simulink model "fukt_test"  (R2023b)
settings: Solver=FixedStepAuto  StartTime=0.0  StopTime=inf  FixedStep=0.5  MaxStep=1  MinStep=1  RelTol=1e-3
undefined symbols (not defined in the file or in its folder): BOOL, DINT, OTL, slplc
libraries: arduinolib x3
(part 3 of 6)

== system fukt_test/PLC Controller Suite/__Logic/Fukt sampling/Fuktmätare sampling/__Logic/Variable Read ==
  __CoreVarRead : Subsystem  Tag=CoreVarReadBlock  DisableCoverage=on  TreatAsAtomicUnit=on  mask{PLCBlockType=CoreVarRead}
      mask init:
      | slplc.callbacks.initCoreVariable(gcb, 'read');
      mask Help: web([docroot '/plccoder/ref/__corevarread' '.html']);
      mask DialogControl PLCBlockTitle Prompt: Core Variable Read
  __Format : MATLAB Function  Tag=PLC_Format_Data  Priority=20  DisableCoverage=on  InitFcn=slplc.utils.setBlockAppearance('reset');  StopFcn=slplc.utils.setBlockAppearance('reset');  TreatAsAtomicUnit=on
  VarOut : Outport  VectorParamsAs1DForOutWhenUnconnected=off
  wires:
  __CoreVarRead/1(y) -> __Format/1(data), VarOut/1

== system fukt_test/PLC Controller Suite/__Logic/Fukt sampling/Fuktmätare sampling/__Logic/Variable Write ==
  VarIn : Inport
  VariableWriteEnableRead : Subsystem  DisableCoverage=on  TreatAsAtomicUnit=on  mask{PLCLabelTag=_Variable_Write_Enable, PLCBlockType=VariableWriteEnableRead}
      mask prompts: PLCLabelTag "Label Tag:"
      mask init:
      | block = gcb;
      | maskObj = Simulink.Mask.get(block);
      | maskObj.Display = sprintf('disp(''%s'');', PLCLabelTag);
      mask Help: web([docroot '/plccoder/ref/variablewriteenableread' '.html']);
      mask DialogControl PLCBlockTitle Prompt: Variable Write Enable Read
      mask Display: disp('_Variable_Write_Enable');
  __CoreVarRead : Subsystem  Tag=CoreVarReadBlock  DisableCoverage=on  TreatAsAtomicUnit=on  mask{PLCBlockType=CoreVarRead}
      mask init:
      | slplc.callbacks.initCoreVariable(gcb, 'read');
      mask Help: web([docroot '/plccoder/ref/__corevarread' '.html']);
      mask DialogControl PLCBlockTitle Prompt: Core Variable Read
  __Enable : Subsystem  Priority=12
  __Format : MATLAB Function  Tag=PLC_Format_Data  Priority=20  DisableCoverage=on  InitFcn=slplc.utils.setBlockAppearance('reset');  StopFcn=slplc.utils.setBlockAppearance('reset');  TreatAsAtomicUnit=on
  wires:
  VarIn/1 -> __Enable/1(VarIn)
  VariableWriteEnableRead/1(Out1) -> __Enable/Enable
  __CoreVarRead/1(y) -> __Format/1(data)

== system fukt_test/PLC Controller Suite/__Logic/Fukt sampling/Fuktmätare sampling/__Logic/XIC1 ==
  RungIn : Inport  PortDimensions=1
  BlockEnableRead : Subsystem  DisableCoverage=on  TreatAsAtomicUnit=on  mask{PLCLabelTag=_Block_Enable, PLCBlockType=BlockEnableRead}
      mask prompts: PLCLabelTag "Label Tag:"
      mask init:
      | block = gcb;
      | maskObj = Simulink.Mask.get(block);
      | maskObj.Display = sprintf('disp(''%s'');', PLCLabelTag);
      mask Help: web([docroot '/plccoder/ref/blockenableread' '.html']);
      mask DialogControl PLCBlockTitle Prompt: Block Enable Read
      mask Display: disp('_Block_Enable');
  Instruction_Enable : Subsystem  Priority=12  TreatAsAtomicUnit=on
  RungInOverride : Subsystem  DisableCoverage=on  TreatAsAtomicUnit=on
  __CoreVarRead : Subsystem  Tag=CoreVarReadBlock  DisableCoverage=on  TreatAsAtomicUnit=on  mask{PLCBlockType=CoreVarRead}
      mask init:
      | slplc.callbacks.initCoreVariable(gcb, 'read');
      mask Help: web([docroot '/plccoder/ref/__corevarread' '.html']);
      mask DialogControl PLCBlockTitle Prompt: Core Variable Read
  __Format : MATLAB Function  Tag=PLC_Format_Boolean  Priority=20  DisableCoverage=on  InitFcn=slplc.utils.setBlockAppearance('reset', '%<PLCOperandTag>');  StopFcn=slplc.utils.setBlockAppearance('reset', '%<PLCOperandTag>');  TreatAsAtomicUnit=on
  RungOut : Outport  OutDataTypeStr=BOOL  PortDimensions=1  InitialOutput=false  VectorParamsAs1DForOutWhenUnconnected=off
  wires:
  RungIn/1 -> RungInOverride/1(In1)
  Instruction_Enable/1(Rung-condition-out) -> __Format/3(RungOut), RungOut/1
  BlockEnableRead/1(Out1) -> __Format/1(BlockEnable), Instruction_Enable/Enable
  RungInOverride/1(Out1) -> __Format/2(RungIn), Instruction_Enable/1(Rung-condition-in)
  __CoreVarRead/1(y) -> __Format/4(data)  "DataBit"

== system fukt_test/PLC Controller Suite/__Logic/Fukt sampling/Fuktmätare sampling/__Logic/XIC2 ==
  RungIn : Inport  PortDimensions=1
  BlockEnableRead : Subsystem  DisableCoverage=on  TreatAsAtomicUnit=on  mask{PLCLabelTag=_Block_Enable, PLCBlockType=BlockEnableRead}
      mask prompts: PLCLabelTag "Label Tag:"
      mask init:
      | block = gcb;
      | maskObj = Simulink.Mask.get(block);
      | maskObj.Display = sprintf('disp(''%s'');', PLCLabelTag);
      mask Help: web([docroot '/plccoder/ref/blockenableread' '.html']);
      mask DialogControl PLCBlockTitle Prompt: Block Enable Read
      mask Display: disp('_Block_Enable');
  Instruction_Enable : Subsystem  Priority=12  TreatAsAtomicUnit=on
  RungInOverride : Subsystem  DisableCoverage=on  TreatAsAtomicUnit=on
  __CoreVarRead : Subsystem  Tag=CoreVarReadBlock  DisableCoverage=on  TreatAsAtomicUnit=on  mask{PLCBlockType=CoreVarRead}
      mask init:
      | slplc.callbacks.initCoreVariable(gcb, 'read');
      mask Help: web([docroot '/plccoder/ref/__corevarread' '.html']);
      mask DialogControl PLCBlockTitle Prompt: Core Variable Read
  __Format : MATLAB Function  Tag=PLC_Format_Boolean  Priority=20  DisableCoverage=on  InitFcn=slplc.utils.setBlockAppearance('reset', '%<PLCOperandTag>');  StopFcn=slplc.utils.setBlockAppearance('reset', '%<PLCOperandTag>');  TreatAsAtomicUnit=on
  RungOut : Outport  OutDataTypeStr=BOOL  PortDimensions=1  InitialOutput=false  VectorParamsAs1DForOutWhenUnconnected=off
  wires:
  __CoreVarRead/1(y) -> __Format/4(data)  "DataBit"
  RungInOverride/1(Out1) -> Instruction_Enable/1(Rung-condition-in), __Format/2(RungIn)
  BlockEnableRead/1(Out1) -> Instruction_Enable/Enable, __Format/1(BlockEnable)
  Instruction_Enable/1(Rung-condition-out) -> RungOut/1, __Format/3(RungOut)
  RungIn/1 -> RungInOverride/1(In1)

== system fukt_test/PLC Controller Suite/__Logic/Fukt logic/Program/__Logic/GEQ/BlockEnableRead ==
  __CoreLabelRead : Subsystem  Tag=CoreVarReadBlock  DisableCoverage=on  TreatAsAtomicUnit=on  mask{PLCBlockType=CoreLabelRead}
      mask init:
      | slplc.callbacks.initRoutineLabelRead(gcb);
      mask Help: web([docroot '/plccoder/ref/__corelabelread' '.html']);
      mask DialogControl PLCBlockTitle Prompt: Core Label Read
  Out1 : Outport  VectorParamsAs1DForOutWhenUnconnected=off
  wires:
  __CoreLabelRead/1(Out1) -> Out1/1

== system fukt_test/PLC Controller Suite/__Logic/Fukt logic/Program/__Logic/GEQ/Instruction_Enable ==
  Rung-condition-in : Inport
  srcA : Inport  Port=2  PortDimensions=1
  srcB : Inport  Port=3  PortDimensions=1
  Enable : EnablePort
  Logical Operator : Logic  OutDataTypeStr=BOOL
  Relational Operator : RelationalOperator  OutDataTypeStr=BOOL  RndMeth=Simplest  InputSameDT=off
  Rung-condition-out : Outport  PortDimensions=1  VectorParamsAs1DForOutWhenUnconnected=off
  wires:
  Rung-condition-in/1 -> Logical Operator/1
  srcB/1 -> Relational Operator/2
  srcA/1 -> Relational Operator/1
  Relational Operator/1 -> Logical Operator/2
  Logical Operator/1 -> Rung-condition-out/1  "Rung-condition-out"

== system fukt_test/PLC Controller Suite/__Logic/Fukt logic/Program/__Logic/GEQ/RungInOverride ==
  In1 : Inport
  AND : Logic  AllPortsSameDT=off  OutDataTypeStr=boolean
  ForceRungInFalseRead : Subsystem  DisableCoverage=on  TreatAsAtomicUnit=on  mask{PLCLabelTag=_Force_RungIn_False, PLCBlockType=ForceRungInFalseRead}
      mask prompts: PLCLabelTag "Label Tag:"
      mask init:
      | block = gcb;
      | maskObj = Simulink.Mask.get(block);
      | maskObj.Display = sprintf('disp(''%s'');', PLCLabelTag);
      mask Help: web([docroot '/plccoder/ref/forcerunginfalseread' '.html']);
      mask DialogControl PLCBlockTitle Prompt: Force Rung-In False Read
      mask Display: disp('_Force_RungIn_False');
  NOT : Logic  Operator=NOT  IconShape=distinctive  AllPortsSameDT=off  OutDataTypeStr=boolean
  Out1 : Outport  VectorParamsAs1DForOutWhenUnconnected=off
  wires:
  AND/1 -> Out1/1
  In1/1 -> AND/2
  ForceRungInFalseRead/1(Out1) -> NOT/1
  NOT/1 -> AND/1

== system fukt_test/PLC Controller Suite/__Logic/Fukt logic/Program/__Logic/OTL/BlockEnableRead ==
  __CoreLabelRead : Subsystem  Tag=CoreVarReadBlock  DisableCoverage=on  TreatAsAtomicUnit=on  mask{PLCBlockType=CoreLabelRead}
      mask init:
      | slplc.callbacks.initRoutineLabelRead(gcb);
      mask Help: web([docroot '/plccoder/ref/__corelabelread' '.html']);
      mask DialogControl PLCBlockTitle Prompt: Core Label Read
  Out1 : Outport  VectorParamsAs1DForOutWhenUnconnected=off
  wires:
  __CoreLabelRead/1(Out1) -> Out1/1

== system fukt_test/PLC Controller Suite/__Logic/Fukt logic/Program/__Logic/OTL/Instruction_Enable ==
  Rung-condition-in : Inport  OutDataTypeStr=BOOL
  Enable : EnablePort
  Rung-condition-in is true : Subsystem  Priority=12
  wires:
  Rung-condition-in/1 -> Rung-condition-in is true/Enable  "Rung-condition-in"

== system fukt_test/PLC Controller Suite/__Logic/Fukt logic/Program/__Logic/OTL/RungInOverride ==
  In1 : Inport
  AND : Logic  AllPortsSameDT=off  OutDataTypeStr=boolean
  ForceRungInFalseRead : Subsystem  DisableCoverage=on  TreatAsAtomicUnit=on  mask{PLCLabelTag=_Force_RungIn_False, PLCBlockType=ForceRungInFalseRead}
      mask prompts: PLCLabelTag "Label Tag:"
      mask init:
      | block = gcb;
      | maskObj = Simulink.Mask.get(block);
      | maskObj.Display = sprintf('disp(''%s'');', PLCLabelTag);
      mask Help: web([docroot '/plccoder/ref/forcerunginfalseread' '.html']);
      mask DialogControl PLCBlockTitle Prompt: Force Rung-In False Read
      mask Display: disp('_Force_RungIn_False');
  NOT : Logic  Operator=NOT  IconShape=distinctive  AllPortsSameDT=off  OutDataTypeStr=boolean
  Out1 : Outport  VectorParamsAs1DForOutWhenUnconnected=off
  wires:
  AND/1 -> Out1/1
  In1/1 -> AND/2
  ForceRungInFalseRead/1(Out1) -> NOT/1
  NOT/1 -> AND/1

== system fukt_test/PLC Controller Suite/__Logic/Fukt logic/Program/__Logic/OTL/__CoreVarRead ==
  DataRead : DataStoreRead  DataStoreName=xxx_PLC_VAR_OrangeLed  IndexOptions=Index vector (dialog)  Indices=1  OutputSizes=1
  y : Outport  VectorParamsAs1DForOutWhenUnconnected=off
  wires:
  DataRead/1 -> y/1

== system fukt_test/PLC Controller Suite/__Logic/Fukt logic/Program/__Logic/OTL1/BlockEnableRead ==
  __CoreLabelRead : Subsystem  Tag=CoreVarReadBlock  DisableCoverage=on  TreatAsAtomicUnit=on  mask{PLCBlockType=CoreLabelRead}
      mask init:
      | slplc.callbacks.initRoutineLabelRead(gcb);
      mask Help: web([docroot '/plccoder/ref/__corelabelread' '.html']);
      mask DialogControl PLCBlockTitle Prompt: Core Label Read
  Out1 : Outport  VectorParamsAs1DForOutWhenUnconnected=off
  wires:
  __CoreLabelRead/1(Out1) -> Out1/1

== system fukt_test/PLC Controller Suite/__Logic/Fukt logic/Program/__Logic/OTL1/Instruction_Enable ==
  Rung-condition-in : Inport  OutDataTypeStr=BOOL
  Enable : EnablePort
  Rung-condition-in is true : Subsystem  Priority=12
  wires:
  Rung-condition-in/1 -> Rung-condition-in is true/Enable  "Rung-condition-in"

== system fukt_test/PLC Controller Suite/__Logic/Fukt logic/Program/__Logic/OTL1/RungInOverride ==
  In1 : Inport
  AND : Logic  AllPortsSameDT=off  OutDataTypeStr=boolean
  ForceRungInFalseRead : Subsystem  DisableCoverage=on  TreatAsAtomicUnit=on  mask{PLCLabelTag=_Force_RungIn_False, PLCBlockType=ForceRungInFalseRead}
      mask prompts: PLCLabelTag "Label Tag:"
      mask init:
      | block = gcb;
      | maskObj = Simulink.Mask.get(block);
      | maskObj.Display = sprintf('disp(''%s'');', PLCLabelTag);
      mask Help: web([docroot '/plccoder/ref/forcerunginfalseread' '.html']);
      mask DialogControl PLCBlockTitle Prompt: Force Rung-In False Read
      mask Display: disp('_Force_RungIn_False');
  NOT : Logic  Operator=NOT  IconShape=distinctive  AllPortsSameDT=off  OutDataTypeStr=boolean
  Out1 : Outport  VectorParamsAs1DForOutWhenUnconnected=off
  wires:
  AND/1 -> Out1/1
  In1/1 -> AND/2
  ForceRungInFalseRead/1(Out1) -> NOT/1
  NOT/1 -> AND/1

== system fukt_test/PLC Controller Suite/__Logic/Fukt logic/Program/__Logic/OTL1/__CoreVarRead ==
  DataRead : DataStoreRead  DataStoreName=xxx_PLC_VAR_fukt_bool  IndexOptions=Index vector (dialog)  Indices=1  OutputSizes=1
  y : Outport  VectorParamsAs1DForOutWhenUnconnected=off
  wires:
  DataRead/1 -> y/1

== system fukt_test/PLC Controller Suite/__Logic/Fukt logic/Program/__Logic/OTU/BlockEnableRead ==
  __CoreLabelRead : Subsystem  Tag=CoreVarReadBlock  DisableCoverage=on  TreatAsAtomicUnit=on  mask{PLCBlockType=CoreLabelRead}
      mask init:
      | slplc.callbacks.initRoutineLabelRead(gcb);
      mask Help: web([docroot '/plccoder/ref/__corelabelread' '.html']);
      mask DialogControl PLCBlockTitle Prompt: Core Label Read
  Out1 : Outport  VectorParamsAs1DForOutWhenUnconnected=off
  wires:
  __CoreLabelRead/1(Out1) -> Out1/1

== system fukt_test/PLC Controller Suite/__Logic/Fukt logic/Program/__Logic/OTU/Instruction_Enable ==
  Rung-condition-in : Inport  OutDataTypeStr=BOOL
  Enable : EnablePort
  Rung-condition-in is true : Subsystem  Priority=12
  wires:
  Rung-condition-in/1 -> Rung-condition-in is true/Enable  "Rung-condition-in"

== system fukt_test/PLC Controller Suite/__Logic/Fukt logic/Program/__Logic/OTU/RungInOverride ==
  In1 : Inport
  AND : Logic  AllPortsSameDT=off  OutDataTypeStr=boolean
  ForceRungInFalseRead : Subsystem  DisableCoverage=on  TreatAsAtomicUnit=on  mask{PLCLabelTag=_Force_RungIn_False, PLCBlockType=ForceRungInFalseRead}
      mask prompts: PLCLabelTag "Label Tag:"
      mask init:
      | block = gcb;
      | maskObj = Simulink.Mask.get(block);
      | maskObj.Display = sprintf('disp(''%s'');', PLCLabelTag);
      mask Help: web([docroot '/plccoder/ref/forcerunginfalseread' '.html']);
      mask DialogControl PLCBlockTitle Prompt: Force Rung-In False Read
      mask Display: disp('_Force_RungIn_False');
  NOT : Logic  Operator=NOT  IconShape=distinctive  AllPortsSameDT=off  OutDataTypeStr=boolean
  Out1 : Outport  VectorParamsAs1DForOutWhenUnconnected=off
  wires:
  AND/1 -> Out1/1
  In1/1 -> AND/2
  ForceRungInFalseRead/1(Out1) -> NOT/1
  NOT/1 -> AND/1

== system fukt_test/PLC Controller Suite/__Logic/Fukt logic/Program/__Logic/OTU/__CoreVarRead ==
  DataRead : DataStoreRead  DataStoreName=xxx_PLC_VAR_OrangeLed  IndexOptions=Index vector (dialog)  Indices=1  OutputSizes=1
  y : Outport  VectorParamsAs1DForOutWhenUnconnected=off
  wires:
  DataRead/1 -> y/1

== system fukt_test/PLC Controller Suite/__Logic/Fukt logic/Program/__Logic/OTU1/BlockEnableRead ==
  __CoreLabelRead : Subsystem  Tag=CoreVarReadBlock  DisableCoverage=on  TreatAsAtomicUnit=on  mask{PLCBlockType=CoreLabelRead}
      mask init:
      | slplc.callbacks.initRoutineLabelRead(gcb);
      mask Help: web([docroot '/plccoder/ref/__corelabelread' '.html']);
      mask DialogControl PLCBlockTitle Prompt: Core Label Read
  Out1 : Outport  VectorParamsAs1DForOutWhenUnconnected=off
  wires:
  __CoreLabelRead/1(Out1) -> Out1/1

== system fukt_test/PLC Controller Suite/__Logic/Fukt logic/Program/__Logic/OTU1/Instruction_Enable ==
  Rung-condition-in : Inport  OutDataTypeStr=BOOL
  Enable : EnablePort
  Rung-condition-in is true : Subsystem  Priority=12
  wires:
  Rung-condition-in/1 -> Rung-condition-in is true/Enable  "Rung-condition-in"

== system fukt_test/PLC Controller Suite/__Logic/Fukt logic/Program/__Logic/OTU1/RungInOverride ==
  In1 : Inport
  AND : Logic  AllPortsSameDT=off  OutDataTypeStr=boolean
  ForceRungInFalseRead : Subsystem  DisableCoverage=on  TreatAsAtomicUnit=on  mask{PLCLabelTag=_Force_RungIn_False, PLCBlockType=ForceRungInFalseRead}
      mask prompts: PLCLabelTag "Label Tag:"
      mask init:
      | block = gcb;
      | maskObj = Simulink.Mask.get(block);
      | maskObj.Display = sprintf('disp(''%s'');', PLCLabelTag);
      mask Help: web([docroot '/plccoder/ref/forcerunginfalseread' '.html']);
      mask DialogControl PLCBlockTitle Prompt: Force Rung-In False Read
      mask Display: disp('_Force_RungIn_False');
  NOT : Logic  Operator=NOT  IconShape=distinctive  AllPortsSameDT=off  OutDataTypeStr=boolean
  Out1 : Outport  VectorParamsAs1DForOutWhenUnconnected=off
  wires:
  AND/1 -> Out1/1
  In1/1 -> AND/2
  ForceRungInFalseRead/1(Out1) -> NOT/1
  NOT/1 -> AND/1

== system fukt_test/PLC Controller Suite/__Logic/Fukt logic/Program/__Logic/OTU1/__CoreVarRead ==
  DataRead : DataStoreRead  DataStoreName=xxx_PLC_VAR_fukt_polling  IndexOptions=Index vector (dialog)  Indices=1  OutputSizes=1
  y : Outport  VectorParamsAs1DForOutWhenUnconnected=off
  wires:
  DataRead/1 -> y/1

== system fukt_test/PLC Controller Suite/__Logic/Fukt logic/Program/__Logic/OTU2/BlockEnableRead ==
  __CoreLabelRead : Subsystem  Tag=CoreVarReadBlock  DisableCoverage=on  TreatAsAtomicUnit=on  mask{PLCBlockType=CoreLabelRead}
      mask init:
      | slplc.callbacks.initRoutineLabelRead(gcb);
      mask Help: web([docroot '/plccoder/ref/__corelabelread' '.html']);
      mask DialogControl PLCBlockTitle Prompt: Core Label Read
  Out1 : Outport  VectorParamsAs1DForOutWhenUnconnected=off
  wires:
  __CoreLabelRead/1(Out1) -> Out1/1

== system fukt_test/PLC Controller Suite/__Logic/Fukt logic/Program/__Logic/OTU2/Instruction_Enable ==
  Rung-condition-in : Inport  OutDataTypeStr=BOOL
  Enable : EnablePort
  Rung-condition-in is true : Subsystem  Priority=12
  wires:
  Rung-condition-in/1 -> Rung-condition-in is true/Enable  "Rung-condition-in"

== system fukt_test/PLC Controller Suite/__Logic/Fukt logic/Program/__Logic/OTU2/RungInOverride ==
  In1 : Inport
  AND : Logic  AllPortsSameDT=off  OutDataTypeStr=boolean
  ForceRungInFalseRead : Subsystem  DisableCoverage=on  TreatAsAtomicUnit=on  mask{PLCLabelTag=_Force_RungIn_False, PLCBlockType=ForceRungInFalseRead}
      mask prompts: PLCLabelTag "Label Tag:"
      mask init:
      | block = gcb;
      | maskObj = Simulink.Mask.get(block);
      | maskObj.Display = sprintf('disp(''%s'');', PLCLabelTag);
      mask Help: web([docroot '/plccoder/ref/forcerunginfalseread' '.html']);
      mask DialogControl PLCBlockTitle Prompt: Force Rung-In False Read
      mask Display: disp('_Force_RungIn_False');
  NOT : Logic  Operator=NOT  IconShape=distinctive  AllPortsSameDT=off  OutDataTypeStr=boolean
  Out1 : Outport  VectorParamsAs1DForOutWhenUnconnected=off
  wires:
  AND/1 -> Out1/1
  In1/1 -> AND/2
  ForceRungInFalseRead/1(Out1) -> NOT/1
  NOT/1 -> AND/1

== system fukt_test/PLC Controller Suite/__Logic/Fukt logic/Program/__Logic/OTU2/__CoreVarRead ==
  DataRead : DataStoreRead  DataStoreName=xxx_PLC_VAR_fukt_bool  IndexOptions=Index vector (dialog)  Indices=1  OutputSizes=1
  y : Outport  VectorParamsAs1DForOutWhenUnconnected=off
  wires:
  DataRead/1 -> y/1

== system fukt_test/PLC Controller Suite/__Logic/Fukt logic/Program/__Logic/TON/BlockEnableRead ==
  __CoreLabelRead : Subsystem  Tag=CoreVarReadBlock  DisableCoverage=on  TreatAsAtomicUnit=on  mask{PLCBlockType=CoreLabelRead}
      mask init:
      | slplc.callbacks.initRoutineLabelRead(gcb);
      mask Help: web([docroot '/plccoder/ref/__corelabelread' '.html']);
      mask DialogControl PLCBlockTitle Prompt: Core Label Read
  Out1 : Outport  VectorParamsAs1DForOutWhenUnconnected=off
  wires:
  __CoreLabelRead/1(Out1) -> Out1/1

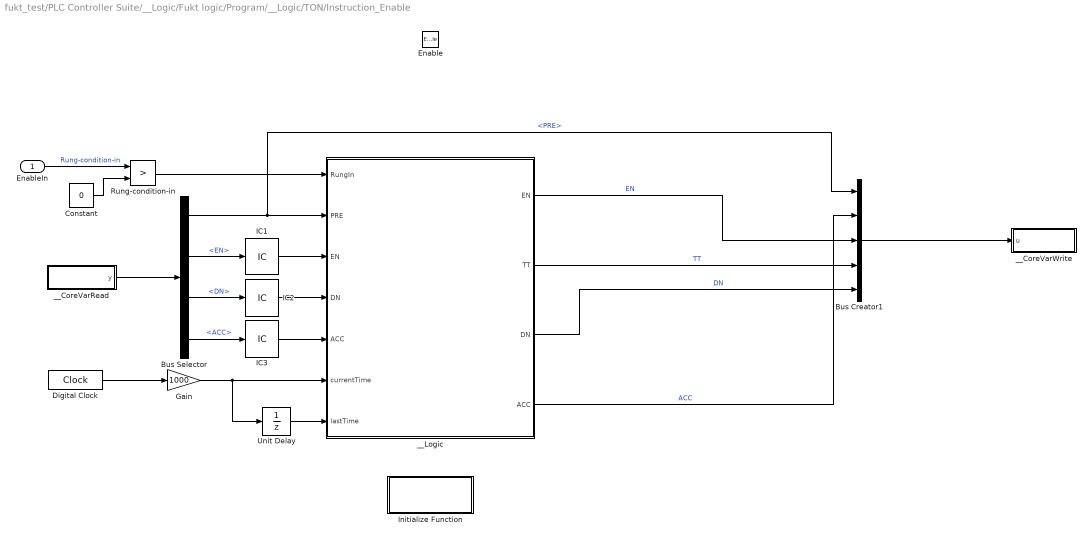
== system fukt_test/PLC Controller Suite/__Logic/Fukt logic/Program/__Logic/TON/Instruction_Enable ==
  EnableIn : Inport
  Enable : EnablePort
  Bus Creator1 : BusCreator  Inputs=5  OutDataTypeStr=Bus: TIMER  NonVirtualBus=on
  Bus Selector : BusSelector  OutputSignals=PRE,EN,DN,ACC
  Constant : Constant  Value=0
  Digital Clock : DigitalClock  SampleTime=PLCTimerSampleTime
  Gain : Gain  Gain=1000
  IC1 : InitialCondition  Value=false
  IC2 : InitialCondition  Value=false
  IC3 : InitialCondition  Value=0
  Initialize Function : Subsystem  TreatAsAtomicUnit=on
  Rung-condition-in : RelationalOperator  Operator=>  OutDataTypeStr=boolean  RndMeth=Simplest  InputSameDT=off
  Unit Delay : UnitDelay  SampleTime=-1  HasFrameUpgradeWarning=on
  __CoreVarRead : Subsystem  Tag=CoreVarReadBlock  DisableCoverage=on  TreatAsAtomicUnit=on  mask{PLCBlockType=CoreVarRead}
      mask init:
      | slplc.callbacks.initCoreVariable(gcb, 'read');
      mask Help: web([docroot '/plccoder/ref/__corevarread' '.html']);
      mask DialogControl PLCBlockTitle Prompt: Core Variable Read
  __CoreVarWrite : Subsystem  Tag=CoreVarWriteBlock  DisableCoverage=on  TreatAsAtomicUnit=on  mask{PLCBlockType=CoreVarWrite}
      mask init:
      | slplc.callbacks.initCoreVariable(gcb, 'write');
      mask Help: web([docroot '/plccoder/ref/__corevarwrite' '.html']);
      mask DialogControl PLCBlockTitle Prompt: Core Variable Write
  __Logic : MATLAB Function  Priority=12  DisableCoverage=on
  wires:
  IC3/1 -> __Logic/5("ACC ")
  IC2/1 -> __Logic/4("DN ")
  IC1/1 -> __Logic/3("EN ")
  Rung-condition-in/1 -> __Logic/1(RungIn)
  Bus Selector/2 -> IC1/1  "<EN>"
  Gain/1 -> __Logic/6(currentTime), Unit Delay/1
  Bus Selector/3 -> IC2/1  "<DN>"
  __CoreVarRead/1(y) -> Bus Selector/1
  Unit Delay/1 -> __Logic/7(lastTime)
  Bus Creator1/1 -> __CoreVarWrite/1(u)
  __Logic/4(ACC) -> Bus Creator1/2  "ACC"
  __Logic/3(DN) -> Bus Creator1/5  "DN"
  Digital Clock/1 -> Gain/1
  EnableIn/1 -> Rung-condition-in/1  "Rung-condition-in"
  Bus Selector/1 -> Bus Creator1/1, __Logic/2(PRE)  "<PRE>"
  __Logic/2(TT) -> Bus Creator1/4  "TT"
  Bus Selector/4 -> IC3/1  "<ACC>"
  __Logic/1(EN) -> Bus Creator1/3  "EN"
  Constant/1 -> Rung-condition-in/2

== system fukt_test/PLC Controller Suite/__Logic/Fukt logic/Program/__Logic/TON/RungInOverride ==
  In1 : Inport
  AND : Logic  AllPortsSameDT=off  OutDataTypeStr=boolean
  ForceRungInFalseRead : Subsystem  DisableCoverage=on  TreatAsAtomicUnit=on  mask{PLCLabelTag=_Force_RungIn_False, PLCBlockType=ForceRungInFalseRead}
      mask prompts: PLCLabelTag "Label Tag:"
      mask init:
      | block = gcb;
      | maskObj = Simulink.Mask.get(block);
      | maskObj.Display = sprintf('disp(''%s'');', PLCLabelTag);
      mask Help: web([docroot '/plccoder/ref/forcerunginfalseread' '.html']);
      mask DialogControl PLCBlockTitle Prompt: Force Rung-In False Read
      mask Display: disp('_Force_RungIn_False');
  NOT : Logic  Operator=NOT  IconShape=distinctive  AllPortsSameDT=off  OutDataTypeStr=boolean
  Out1 : Outport  VectorParamsAs1DForOutWhenUnconnected=off
  wires:
  AND/1 -> Out1/1
  In1/1 -> AND/2
  ForceRungInFalseRead/1(Out1) -> NOT/1
  NOT/1 -> AND/1

== system fukt_test/PLC Controller Suite/__Logic/Fukt logic/Program/__Logic/TON/__CoreVarRead ==
  DataRead : DataStoreRead  DataStoreName=xxx_PLC_VAR_orange_led_timer_1  IndexOptions=Index vector (dialog)  Indices=1  OutputSizes=1
  y : Outport  VectorParamsAs1DForOutWhenUnconnected=off
  wires:
  DataRead/1 -> y/1

== system fukt_test/PLC Controller Suite/__Logic/Fukt logic/Program/__Logic/Variable Read/__CoreVarRead ==
  DataRead : DataStoreRead  DataStoreName=xxx_PLC_VAR_Fukt_value_copy  IndexOptions=Index vector (dialog)  Indices=1  OutputSizes=1
  y : Outport  VectorParamsAs1DForOutWhenUnconnected=off
  wires:
  DataRead/1 -> y/1

== system fukt_test/PLC Controller Suite/__Logic/Fukt logic/Program/__Logic/Variable Read1/__CoreVarRead ==
  DataRead : DataStoreRead  DataStoreName=xxx_PLC_VAR_Fukt_constant  IndexOptions=Index vector (dialog)  Indices=1  OutputSizes=1
  y : Outport  VectorParamsAs1DForOutWhenUnconnected=off
  wires:
  DataRead/1 -> y/1

== system fukt_test/PLC Controller Suite/__Logic/Fukt logic/Program/__Logic/XIC1/BlockEnableRead ==
  __CoreLabelRead : Subsystem  Tag=CoreVarReadBlock  DisableCoverage=on  TreatAsAtomicUnit=on  mask{PLCBlockType=CoreLabelRead}
      mask init:
      | slplc.callbacks.initRoutineLabelRead(gcb);
      mask Help: web([docroot '/plccoder/ref/__corelabelread' '.html']);
      mask DialogControl PLCBlockTitle Prompt: Core Label Read
  Out1 : Outport  VectorParamsAs1DForOutWhenUnconnected=off
  wires:
  __CoreLabelRead/1(Out1) -> Out1/1

== system fukt_test/PLC Controller Suite/__Logic/Fukt logic/Program/__Logic/XIC1/Instruction_Enable ==
  Rung-condition-in : Inport  OutDataTypeStr=BOOL
  Enable : EnablePort
  Logical Operator : Logic  OutDataTypeStr=BOOL
  __CoreVarRead : Subsystem  Tag=CoreVarReadBlock  DisableCoverage=on  TreatAsAtomicUnit=on  mask{PLCBlockType=CoreVarRead}
      mask init:
      | slplc.callbacks.initCoreVariable(gcb, 'read');
      mask Help: web([docroot '/plccoder/ref/__corevarread' '.html']);
      mask DialogControl PLCBlockTitle Prompt: Core Variable Read
  Rung-condition-out : Outport  VectorParamsAs1DForOutWhenUnconnected=off
  wires:
  Rung-condition-in/1 -> Logical Operator/1  "Rung-condition-in"
  Logical Operator/1 -> Rung-condition-out/1  "Rung-condition-out"
  __CoreVarRead/1(y) -> Logical Operator/2  "DataBit"

== system fukt_test/PLC Controller Suite/__Logic/Fukt logic/Program/__Logic/XIC1/RungInOverride ==
  In1 : Inport
  AND : Logic  AllPortsSameDT=off  OutDataTypeStr=boolean
  ForceRungInFalseRead : Subsystem  DisableCoverage=on  TreatAsAtomicUnit=on  mask{PLCLabelTag=_Force_RungIn_False, PLCBlockType=ForceRungInFalseRead}
      mask prompts: PLCLabelTag "Label Tag:"
      mask init:
      | block = gcb;
      | maskObj = Simulink.Mask.get(block);
      | maskObj.Display = sprintf('disp(''%s'');', PLCLabelTag);
      mask Help: web([docroot '/plccoder/ref/forcerunginfalseread' '.html']);
      mask DialogControl PLCBlockTitle Prompt: Force Rung-In False Read
      mask Display: disp('_Force_RungIn_False');
  NOT : Logic  Operator=NOT  IconShape=distinctive  AllPortsSameDT=off  OutDataTypeStr=boolean
  Out1 : Outport  VectorParamsAs1DForOutWhenUnconnected=off
  wires:
  AND/1 -> Out1/1
  In1/1 -> AND/2
  ForceRungInFalseRead/1(Out1) -> NOT/1
  NOT/1 -> AND/1

== system fukt_test/PLC Controller Suite/__Logic/Fukt logic/Program/__Logic/XIC1/__CoreVarRead ==
  DataRead : DataStoreRead  DataStoreName=xxx_PLC_VAR_orange_led_timer_1  DataStoreElements=xxx_PLC_VAR_orange_led_timer_1.DN  IndexOptions=Index vector (dialog)  Indices=1  OutputSizes=1
  y : Outport  VectorParamsAs1DForOutWhenUnconnected=off
  wires:
  DataRead/1 -> y/1

== system fukt_test/PLC Controller Suite/__Logic/Fukt logic/Program/__Logic/XIC2/BlockEnableRead ==
  __CoreLabelRead : Subsystem  Tag=CoreVarReadBlock  DisableCoverage=on  TreatAsAtomicUnit=on  mask{PLCBlockType=CoreLabelRead}
      mask init:
      | slplc.callbacks.initRoutineLabelRead(gcb);
      mask Help: web([docroot '/plccoder/ref/__corelabelread' '.html']);
      mask DialogControl PLCBlockTitle Prompt: Core Label Read
  Out1 : Outport  VectorParamsAs1DForOutWhenUnconnected=off
  wires:
  __CoreLabelRead/1(Out1) -> Out1/1

== system fukt_test/PLC Controller Suite/__Logic/Fukt logic/Program/__Logic/XIC2/Instruction_Enable ==
  Rung-condition-in : Inport  OutDataTypeStr=BOOL
  Enable : EnablePort
  Logical Operator : Logic  OutDataTypeStr=BOOL
  __CoreVarRead : Subsystem  Tag=CoreVarReadBlock  DisableCoverage=on  TreatAsAtomicUnit=on  mask{PLCBlockType=CoreVarRead}
      mask init:
      | slplc.callbacks.initCoreVariable(gcb, 'read');
      mask Help: web([docroot '/plccoder/ref/__corevarread' '.html']);
      mask DialogControl PLCBlockTitle Prompt: Core Variable Read
  Rung-condition-out : Outport  VectorParamsAs1DForOutWhenUnconnected=off
  wires:
  __CoreVarRead/1(y) -> Logical Operator/2  "DataBit"
  Logical Operator/1 -> Rung-condition-out/1  "Rung-condition-out"
  Rung-condition-in/1 -> Logical Operator/1  "Rung-condition-in"

== system fukt_test/PLC Controller Suite/__Logic/Fukt logic/Program/__Logic/XIC2/RungInOverride ==
  In1 : Inport
  AND : Logic  AllPortsSameDT=off  OutDataTypeStr=boolean
  ForceRungInFalseRead : Subsystem  DisableCoverage=on  TreatAsAtomicUnit=on  mask{PLCLabelTag=_Force_RungIn_False, PLCBlockType=ForceRungInFalseRead}
      mask prompts: PLCLabelTag "Label Tag:"
      mask init:
      | block = gcb;
      | maskObj = Simulink.Mask.get(block);
      | maskObj.Display = sprintf('disp(''%s'');', PLCLabelTag);
      mask Help: web([docroot '/plccoder/ref/forcerunginfalseread' '.html']);
      mask DialogControl PLCBlockTitle Prompt: Force Rung-In False Read
      mask Display: disp('_Force_RungIn_False');
  NOT : Logic  Operator=NOT  IconShape=distinctive  AllPortsSameDT=off  OutDataTypeStr=boolean
  Out1 : Outport  VectorParamsAs1DForOutWhenUnconnected=off
  wires:
  NOT/1 -> AND/1
  ForceRungInFalseRead/1(Out1) -> NOT/1
  In1/1 -> AND/2
  AND/1 -> Out1/1

== system fukt_test/PLC Controller Suite/__Logic/Fukt logic/Program/__Logic/XIC2/__CoreVarRead ==
  DataRead : DataStoreRead  DataStoreName=xxx_PLC_VAR_fukt_polling  IndexOptions=Index vector (dialog)  Indices=1  OutputSizes=1
  y : Outport  VectorParamsAs1DForOutWhenUnconnected=off
  wires:
  DataRead/1 -> y/1

== system fukt_test/PLC Controller Suite/__Logic/Fukt logic/Program/__Logic/XIC3/BlockEnableRead ==
  __CoreLabelRead : Subsystem  Tag=CoreVarReadBlock  DisableCoverage=on  TreatAsAtomicUnit=on  mask{PLCBlockType=CoreLabelRead}
      mask init:
      | slplc.callbacks.initRoutineLabelRead(gcb);
      mask Help: web([docroot '/plccoder/ref/__corelabelread' '.html']);
      mask DialogControl PLCBlockTitle Prompt: Core Label Read
  Out1 : Outport  VectorParamsAs1DForOutWhenUnconnected=off
  wires:
  __CoreLabelRead/1(Out1) -> Out1/1

== system fukt_test/PLC Controller Suite/__Logic/Fukt logic/Program/__Logic/XIC3/Instruction_Enable ==
  Rung-condition-in : Inport  OutDataTypeStr=BOOL
  Enable : EnablePort
  Logical Operator : Logic  OutDataTypeStr=BOOL
  __CoreVarRead : Subsystem  Tag=CoreVarReadBlock  DisableCoverage=on  TreatAsAtomicUnit=on  mask{PLCBlockType=CoreVarRead}
      mask init:
      | slplc.callbacks.initCoreVariable(gcb, 'read');
      mask Help: web([docroot '/plccoder/ref/__corevarread' '.html']);
      mask DialogControl PLCBlockTitle Prompt: Core Variable Read
  Rung-condition-out : Outport  VectorParamsAs1DForOutWhenUnconnected=off
  wires:
  Rung-condition-in/1 -> Logical Operator/1  "Rung-condition-in"
  Logical Operator/1 -> Rung-condition-out/1  "Rung-condition-out"
  __CoreVarRead/1(y) -> Logical Operator/2  "DataBit"

== system fukt_test/PLC Controller Suite/__Logic/Fukt logic/Program/__Logic/XIC3/RungInOverride ==
  In1 : Inport
  AND : Logic  AllPortsSameDT=off  OutDataTypeStr=boolean
  ForceRungInFalseRead : Subsystem  DisableCoverage=on  TreatAsAtomicUnit=on  mask{PLCLabelTag=_Force_RungIn_False, PLCBlockType=ForceRungInFalseRead}
      mask prompts: PLCLabelTag "Label Tag:"
      mask init:
      | block = gcb;
      | maskObj = Simulink.Mask.get(block);
      | maskObj.Display = sprintf('disp(''%s'');', PLCLabelTag);
      mask Help: web([docroot '/plccoder/ref/forcerunginfalseread' '.html']);
      mask DialogControl PLCBlockTitle Prompt: Force Rung-In False Read
      mask Display: disp('_Force_RungIn_False');
  NOT : Logic  Operator=NOT  IconShape=distinctive  AllPortsSameDT=off  OutDataTypeStr=boolean
  Out1 : Outport  VectorParamsAs1DForOutWhenUnconnected=off
  wires:
  AND/1 -> Out1/1
  In1/1 -> AND/2
  ForceRungInFalseRead/1(Out1) -> NOT/1
  NOT/1 -> AND/1

== system fukt_test/PLC Controller Suite/__Logic/Fukt logic/Program/__Logic/XIC3/__CoreVarRead ==
  DataRead : DataStoreRead  DataStoreName=xxx_PLC_VAR_fukt_bool  IndexOptions=Index vector (dialog)  Indices=1  OutputSizes=1
  y : Outport  VectorParamsAs1DForOutWhenUnconnected=off
  wires:
  DataRead/1 -> y/1

== system fukt_test/PLC Controller Suite/__Logic/Fukt sampling/Fuktmätare sampling/__Logic/MOV/BlockEnableRead ==
  __CoreLabelRead : Subsystem  Tag=CoreVarReadBlock  DisableCoverage=on  TreatAsAtomicUnit=on  mask{PLCBlockType=CoreLabelRead}
      mask init:
      | slplc.callbacks.initRoutineLabelRead(gcb);
      mask Help: web([docroot '/plccoder/ref/__corelabelread' '.html']);
      mask DialogControl PLCBlockTitle Prompt: Core Label Read
  Out1 : Outport  VectorParamsAs1DForOutWhenUnconnected=off
  wires:
  __CoreLabelRead/1(Out1) -> Out1/1

== system fukt_test/PLC Controller Suite/__Logic/Fukt sampling/Fuktmätare sampling/__Logic/MOV/Instruction_Enable ==
  src : Inport  PortDimensions=1
  Enable : EnablePort
  Data Type Conversion : DataTypeConversion  RndMeth=Convergent  SaturateOnIntegerOverflow=off
  dest : Outport  PortDimensions=1  VectorParamsAs1DForOutWhenUnconnected=off
  wires:
  Data Type Conversion/1 -> dest/1
  src/1 -> Data Type Conversion/1

== system fukt_test/PLC Controller Suite/__Logic/Fukt sampling/Fuktmätare sampling/__Logic/MOV/RungInOverride ==
  In1 : Inport
  AND : Logic  AllPortsSameDT=off  OutDataTypeStr=boolean
  ForceRungInFalseRead : Subsystem  DisableCoverage=on  TreatAsAtomicUnit=on  mask{PLCLabelTag=_Force_RungIn_False, PLCBlockType=ForceRungInFalseRead}
      mask prompts: PLCLabelTag "Label Tag:"
      mask init:
      | block = gcb;
      | maskObj = Simulink.Mask.get(block);
      | maskObj.Display = sprintf('disp(''%s'');', PLCLabelTag);
      mask Help: web([docroot '/plccoder/ref/forcerunginfalseread' '.html']);
      mask DialogControl PLCBlockTitle Prompt: Force Rung-In False Read
      mask Display: disp('_Force_RungIn_False');
  NOT : Logic  Operator=NOT  IconShape=distinctive  AllPortsSameDT=off  OutDataTypeStr=boolean
  Out1 : Outport  VectorParamsAs1DForOutWhenUnconnected=off
  wires:
  AND/1 -> Out1/1
  In1/1 -> AND/2
  ForceRungInFalseRead/1(Out1) -> NOT/1
  NOT/1 -> AND/1

== system fukt_test/PLC Controller Suite/__Logic/Fukt sampling/Fuktmätare sampling/__Logic/MOV/RungOutOverride ==
  In1 : Inport
  AND : Logic  AllPortsSameDT=off  OutDataTypeStr=boolean
  BlockEnableRead : Subsystem  DisableCoverage=on  TreatAsAtomicUnit=on  mask{PLCLabelTag=_Block_Enable, PLCBlockType=BlockEnableRead}
      mask prompts: PLCLabelTag "Label Tag:"
      mask init:
      | block = gcb;
      | maskObj = Simulink.Mask.get(block);
      | maskObj.Display = sprintf('disp(''%s'');', PLCLabelTag);
      mask Help: web([docroot '/plccoder/ref/blockenableread' '.html']);
      mask DialogControl PLCBlockTitle Prompt: Block Enable Read
      mask Display: disp('_Block_Enable');
  VariableWriteEnableWrite : Subsystem  DisableCoverage=on  TreatAsAtomicUnit=on  mask{PLCLabelTag=_Variable_Write_Enable, PLCBlockType=VariableWriteEnableWrite}
      mask prompts: PLCLabelTag "Label Tag:"
      mask init:
      | block = gcb;
      | maskObj = Simulink.Mask.get(block);
      | maskObj.Display = sprintf('disp(''%s'');', PLCLabelTag);
      mask Help: web([docroot '/plccoder/ref/variablewriteenablewrite' '.html']);
      mask DialogControl PLCBlockTitle Prompt: Variable Write_Enable_Write
      mask Display: disp('_Variable_Write_Enable');
  Out1 : Outport  VectorParamsAs1DForOutWhenUnconnected=off
  wires:
  AND/1 -> VariableWriteEnableWrite/1(In1), Out1/1
  BlockEnableRead/1(Out1) -> AND/1
  In1/1 -> AND/2

== system fukt_test/PLC Controller Suite/__Logic/Fukt sampling/Fuktmätare sampling/__Logic/OTL/BlockEnableRead ==
  __CoreLabelRead : Subsystem  Tag=CoreVarReadBlock  DisableCoverage=on  TreatAsAtomicUnit=on  mask{PLCBlockType=CoreLabelRead}
      mask init:
      | slplc.callbacks.initRoutineLabelRead(gcb);
      mask Help: web([docroot '/plccoder/ref/__corelabelread' '.html']);
      mask DialogControl PLCBlockTitle Prompt: Core Label Read
  Out1 : Outport  VectorParamsAs1DForOutWhenUnconnected=off
  wires:
  __CoreLabelRead/1(Out1) -> Out1/1

== system fukt_test/PLC Controller Suite/__Logic/Fukt sampling/Fuktmätare sampling/__Logic/OTL/Instruction_Enable ==
  Rung-condition-in : Inport  OutDataTypeStr=BOOL
  Enable : EnablePort
  Rung-condition-in is true : Subsystem  Priority=12
  wires:
  Rung-condition-in/1 -> Rung-condition-in is true/Enable  "Rung-condition-in"

== system fukt_test/PLC Controller Suite/__Logic/Fukt sampling/Fuktmätare sampling/__Logic/OTL/RungInOverride ==
  In1 : Inport
  AND : Logic  AllPortsSameDT=off  OutDataTypeStr=boolean
  ForceRungInFalseRead : Subsystem  DisableCoverage=on  TreatAsAtomicUnit=on  mask{PLCLabelTag=_Force_RungIn_False, PLCBlockType=ForceRungInFalseRead}
      mask prompts: PLCLabelTag "Label Tag:"
      mask init:
      | block = gcb;
      | maskObj = Simulink.Mask.get(block);
      | maskObj.Display = sprintf('disp(''%s'');', PLCLabelTag);
      mask Help: web([docroot '/plccoder/ref/forcerunginfalseread' '.html']);
      mask DialogControl PLCBlockTitle Prompt: Force Rung-In False Read
      mask Display: disp('_Force_RungIn_False');
  NOT : Logic  Operator=NOT  IconShape=distinctive  AllPortsSameDT=off  OutDataTypeStr=boolean
  Out1 : Outport  VectorParamsAs1DForOutWhenUnconnected=off
  wires:
  AND/1 -> Out1/1
  In1/1 -> AND/2
  ForceRungInFalseRead/1(Out1) -> NOT/1
  NOT/1 -> AND/1

== system fukt_test/PLC Controller Suite/__Logic/Fukt sampling/Fuktmätare sampling/__Logic/OTL/__CoreVarRead ==
  DataRead : DataStoreRead  DataStoreName=xxx_PLC_VAR_fukt_polling  IndexOptions=Index vector (dialog)  Indices=1  OutputSizes=1
  y : Outport  VectorParamsAs1DForOutWhenUnconnected=off
  wires:
  DataRead/1 -> y/1

== system fukt_test/PLC Controller Suite/__Logic/Fukt sampling/Fuktmätare sampling/__Logic/OTL1/BlockEnableRead ==
  __CoreLabelRead : Subsystem  Tag=CoreVarReadBlock  DisableCoverage=on  TreatAsAtomicUnit=on  mask{PLCBlockType=CoreLabelRead}
      mask init:
      | slplc.callbacks.initRoutineLabelRead(gcb);
      mask Help: web([docroot '/plccoder/ref/__corelabelread' '.html']);
      mask DialogControl PLCBlockTitle Prompt: Core Label Read
  Out1 : Outport  VectorParamsAs1DForOutWhenUnconnected=off
  wires:
  __CoreLabelRead/1(Out1) -> Out1/1

== system fukt_test/PLC Controller Suite/__Logic/Fukt sampling/Fuktmätare sampling/__Logic/OTL1/Instruction_Enable ==
  Rung-condition-in : Inport  OutDataTypeStr=BOOL
  Enable : EnablePort
  Rung-condition-in is true : Subsystem  Priority=12
  wires:
  Rung-condition-in/1 -> Rung-condition-in is true/Enable  "Rung-condition-in"

== system fukt_test/PLC Controller Suite/__Logic/Fukt sampling/Fuktmätare sampling/__Logic/OTL1/RungInOverride ==
  In1 : Inport
  AND : Logic  AllPortsSameDT=off  OutDataTypeStr=boolean
  ForceRungInFalseRead : Subsystem  DisableCoverage=on  TreatAsAtomicUnit=on  mask{PLCLabelTag=_Force_RungIn_False, PLCBlockType=ForceRungInFalseRead}
      mask prompts: PLCLabelTag "Label Tag:"
      mask init:
      | block = gcb;
      | maskObj = Simulink.Mask.get(block);
      | maskObj.Display = sprintf('disp(''%s'');', PLCLabelTag);
      mask Help: web([docroot '/plccoder/ref/forcerunginfalseread' '.html']);
      mask DialogControl PLCBlockTitle Prompt: Force Rung-In False Read
      mask Display: disp('_Force_RungIn_False');
  NOT : Logic  Operator=NOT  IconShape=distinctive  AllPortsSameDT=off  OutDataTypeStr=boolean
  Out1 : Outport  VectorParamsAs1DForOutWhenUnconnected=off
  wires:
  AND/1 -> Out1/1
  In1/1 -> AND/2
  ForceRungInFalseRead/1(Out1) -> NOT/1
  NOT/1 -> AND/1

== system fukt_test/PLC Controller Suite/__Logic/Fukt sampling/Fuktmätare sampling/__Logic/OTL1/__CoreVarRead ==
  DataRead : DataStoreRead  DataStoreName=xxx_PLC_VAR_fukt_power  IndexOptions=Index vector (dialog)  Indices=1  OutputSizes=1
  y : Outport  VectorParamsAs1DForOutWhenUnconnected=off
  wires:
  DataRead/1 -> y/1

== system fukt_test/PLC Controller Suite/__Logic/Fukt sampling/Fuktmätare sampling/__Logic/OTU/BlockEnableRead ==
  __CoreLabelRead : Subsystem  Tag=CoreVarReadBlock  DisableCoverage=on  TreatAsAtomicUnit=on  mask{PLCBlockType=CoreLabelRead}
      mask init:
      | slplc.callbacks.initRoutineLabelRead(gcb);
      mask Help: web([docroot '/plccoder/ref/__corelabelread' '.html']);
      mask DialogControl PLCBlockTitle Prompt: Core Label Read
  Out1 : Outport  VectorParamsAs1DForOutWhenUnconnected=off
  wires:
  __CoreLabelRead/1(Out1) -> Out1/1

== system fukt_test/PLC Controller Suite/__Logic/Fukt sampling/Fuktmätare sampling/__Logic/OTU/Instruction_Enable ==
  Rung-condition-in : Inport  OutDataTypeStr=BOOL
  Enable : EnablePort
  Rung-condition-in is true : Subsystem  Priority=12
  wires:
  Rung-condition-in/1 -> Rung-condition-in is true/Enable  "Rung-condition-in"

== system fukt_test/PLC Controller Suite/__Logic/Fukt sampling/Fuktmätare sampling/__Logic/OTU/RungInOverride ==
  In1 : Inport
  AND : Logic  AllPortsSameDT=off  OutDataTypeStr=boolean
  ForceRungInFalseRead : Subsystem  DisableCoverage=on  TreatAsAtomicUnit=on  mask{PLCLabelTag=_Force_RungIn_False, PLCBlockType=ForceRungInFalseRead}
      mask prompts: PLCLabelTag "Label Tag:"
      mask init:
      | block = gcb;
      | maskObj = Simulink.Mask.get(block);
      | maskObj.Display = sprintf('disp(''%s'');', PLCLabelTag);
      mask Help: web([docroot '/plccoder/ref/forcerunginfalseread' '.html']);
      mask DialogControl PLCBlockTitle Prompt: Force Rung-In False Read
      mask Display: disp('_Force_RungIn_False');
  NOT : Logic  Operator=NOT  IconShape=distinctive  AllPortsSameDT=off  OutDataTypeStr=boolean
  Out1 : Outport  VectorParamsAs1DForOutWhenUnconnected=off
  wires:
  AND/1 -> Out1/1
  In1/1 -> AND/2
  ForceRungInFalseRead/1(Out1) -> NOT/1
  NOT/1 -> AND/1

== system fukt_test/PLC Controller Suite/__Logic/Fukt sampling/Fuktmätare sampling/__Logic/OTU/__CoreVarRead ==
  DataRead : DataStoreRead  DataStoreName=xxx_PLC_VAR_fukt_power  IndexOptions=Index vector (dialog)  Indices=1  OutputSizes=1
  y : Outport  VectorParamsAs1DForOutWhenUnconnected=off
  wires:
  DataRead/1 -> y/1

== system fukt_test/PLC Controller Suite/__Logic/Fukt sampling/Fuktmätare sampling/__Logic/RES/BlockEnableRead ==
  __CoreLabelRead : Subsystem  Tag=CoreVarReadBlock  DisableCoverage=on  TreatAsAtomicUnit=on  mask{PLCBlockType=CoreLabelRead}
      mask init:
      | slplc.callbacks.initRoutineLabelRead(gcb);
      mask Help: web([docroot '/plccoder/ref/__corelabelread' '.html']);
      mask DialogControl PLCBlockTitle Prompt: Core Label Read
  Out1 : Outport  VectorParamsAs1DForOutWhenUnconnected=off
  wires:
  __CoreLabelRead/1(Out1) -> Out1/1

== system fukt_test/PLC Controller Suite/__Logic/Fukt sampling/Fuktmätare sampling/__Logic/RES/Instruction_Enable ==
  Rung-condition-in : Inport
  Enable : EnablePort
  Rung-condition-in is true : Subsystem  TreatAsAtomicUnit=on
  wires:
  Rung-condition-in/1 -> Rung-condition-in is true/Enable

== system fukt_test/PLC Controller Suite/__Logic/Fukt sampling/Fuktmätare sampling/__Logic/RES/RungInOverride ==
  In1 : Inport
  AND : Logic  AllPortsSameDT=off  OutDataTypeStr=boolean
  ForceRungInFalseRead : Subsystem  DisableCoverage=on  TreatAsAtomicUnit=on  mask{PLCLabelTag=_Force_RungIn_False, PLCBlockType=ForceRungInFalseRead}
      mask prompts: PLCLabelTag "Label Tag:"
      mask init:
      | block = gcb;
      | maskObj = Simulink.Mask.get(block);
      | maskObj.Display = sprintf('disp(''%s'');', PLCLabelTag);
      mask Help: web([docroot '/plccoder/ref/forcerunginfalseread' '.html']);
      mask DialogControl PLCBlockTitle Prompt: Force Rung-In False Read
      mask Display: disp('_Force_RungIn_False');
  NOT : Logic  Operator=NOT  IconShape=distinctive  AllPortsSameDT=off  OutDataTypeStr=boolean
  Out1 : Outport  VectorParamsAs1DForOutWhenUnconnected=off
  wires:
  AND/1 -> Out1/1
  In1/1 -> AND/2
  ForceRungInFalseRead/1(Out1) -> NOT/1
  NOT/1 -> AND/1

== system fukt_test/PLC Controller Suite/__Logic/Fukt sampling/Fuktmätare sampling/__Logic/RES/__CoreVarRead ==
  DataRead : DataStoreRead  DataStoreName=xxx_PLC_VAR_Fukt_periodicity  IndexOptions=Index vector (dialog)  Indices=1  OutputSizes=1
  y : Outport  VectorParamsAs1DForOutWhenUnconnected=off
  wires:
  DataRead/1 -> y/1

== system fukt_test/PLC Controller Suite/__Logic/Fukt sampling/Fuktmätare sampling/__Logic/TON/BlockEnableRead ==
  __CoreLabelRead : Subsystem  Tag=CoreVarReadBlock  DisableCoverage=on  TreatAsAtomicUnit=on  mask{PLCBlockType=CoreLabelRead}
      mask init:
      | slplc.callbacks.initRoutineLabelRead(gcb);
      mask Help: web([docroot '/plccoder/ref/__corelabelread' '.html']);
      mask DialogControl PLCBlockTitle Prompt: Core Label Read
  Out1 : Outport  VectorParamsAs1DForOutWhenUnconnected=off
  wires:
  __CoreLabelRead/1(Out1) -> Out1/1

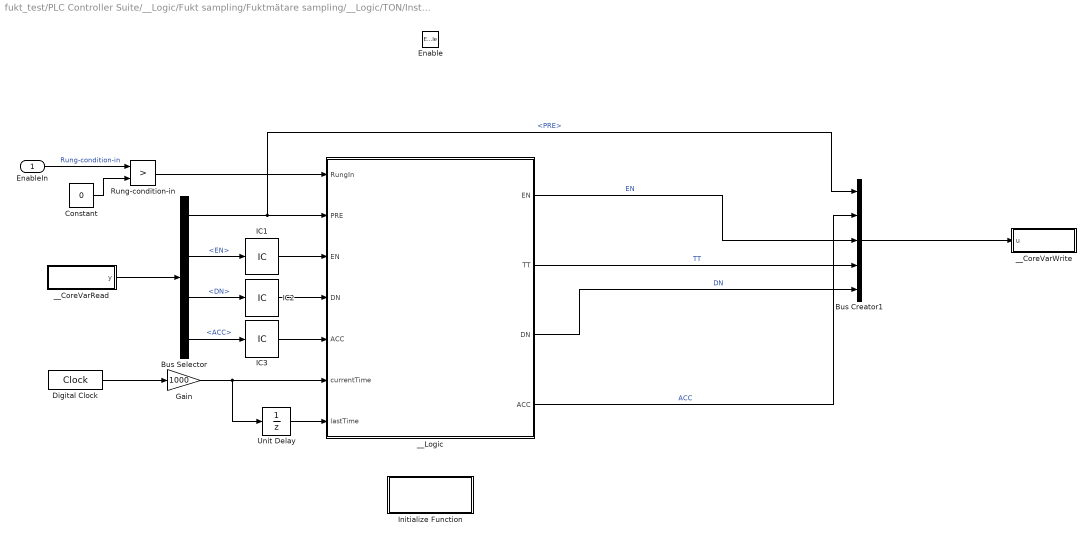
== system fukt_test/PLC Controller Suite/__Logic/Fukt sampling/Fuktmätare sampling/__Logic/TON/Instruction_Enable ==
  EnableIn : Inport
  Enable : EnablePort
  Bus Creator1 : BusCreator  Inputs=5  OutDataTypeStr=Bus: TIMER  NonVirtualBus=on
  Bus Selector : BusSelector  OutputSignals=PRE,EN,DN,ACC
  Constant : Constant  Value=0
  Digital Clock : DigitalClock  SampleTime=PLCTimerSampleTime
  Gain : Gain  Gain=1000
  IC1 : InitialCondition  Value=false
  IC2 : InitialCondition  Value=false
  IC3 : InitialCondition  Value=0
  Initialize Function : Subsystem  TreatAsAtomicUnit=on
  Rung-condition-in : RelationalOperator  Operator=>  OutDataTypeStr=boolean  RndMeth=Simplest  InputSameDT=off
  Unit Delay : UnitDelay  SampleTime=-1  HasFrameUpgradeWarning=on
  __CoreVarRead : Subsystem  Tag=CoreVarReadBlock  DisableCoverage=on  TreatAsAtomicUnit=on  mask{PLCBlockType=CoreVarRead}
      mask init:
      | slplc.callbacks.initCoreVariable(gcb, 'read');
      mask Help: web([docroot '/plccoder/ref/__corevarread' '.html']);
      mask DialogControl PLCBlockTitle Prompt: Core Variable Read
  __CoreVarWrite : Subsystem  Tag=CoreVarWriteBlock  DisableCoverage=on  TreatAsAtomicUnit=on  mask{PLCBlockType=CoreVarWrite}
      mask init:
      | slplc.callbacks.initCoreVariable(gcb, 'write');
      mask Help: web([docroot '/plccoder/ref/__corevarwrite' '.html']);
      mask DialogControl PLCBlockTitle Prompt: Core Variable Write
  __Logic : MATLAB Function  Priority=12  DisableCoverage=on
  wires:
  IC3/1 -> __Logic/5("ACC ")
  IC2/1 -> __Logic/4("DN ")
  IC1/1 -> __Logic/3("EN ")
  Rung-condition-in/1 -> __Logic/1(RungIn)
  Bus Selector/2 -> IC1/1  "<EN>"
  Gain/1 -> __Logic/6(currentTime), Unit Delay/1
  Bus Selector/3 -> IC2/1  "<DN>"
  __CoreVarRead/1(y) -> Bus Selector/1
  Unit Delay/1 -> __Logic/7(lastTime)
  Bus Creator1/1 -> __CoreVarWrite/1(u)
  __Logic/4(ACC) -> Bus Creator1/2  "ACC"
  __Logic/3(DN) -> Bus Creator1/5  "DN"
  Digital Clock/1 -> Gain/1
  EnableIn/1 -> Rung-condition-in/1  "Rung-condition-in"
  Bus Selector/1 -> Bus Creator1/1, __Logic/2(PRE)  "<PRE>"
  __Logic/2(TT) -> Bus Creator1/4  "TT"
  Bus Selector/4 -> IC3/1  "<ACC>"
  __Logic/1(EN) -> Bus Creator1/3  "EN"
  Constant/1 -> Rung-condition-in/2

== system fukt_test/PLC Controller Suite/__Logic/Fukt sampling/Fuktmätare sampling/__Logic/TON/RungInOverride ==
  In1 : Inport
  AND : Logic  AllPortsSameDT=off  OutDataTypeStr=boolean
  ForceRungInFalseRead : Subsystem  DisableCoverage=on  TreatAsAtomicUnit=on  mask{PLCLabelTag=_Force_RungIn_False, PLCBlockType=ForceRungInFalseRead}
      mask prompts: PLCLabelTag "Label Tag:"
      mask init:
      | block = gcb;
      | maskObj = Simulink.Mask.get(block);
      | maskObj.Display = sprintf('disp(''%s'');', PLCLabelTag);
      mask Help: web([docroot '/plccoder/ref/forcerunginfalseread' '.html']);
      mask DialogControl PLCBlockTitle Prompt: Force Rung-In False Read
      mask Display: disp('_Force_RungIn_False');
  NOT : Logic  Operator=NOT  IconShape=distinctive  AllPortsSameDT=off  OutDataTypeStr=boolean
  Out1 : Outport  VectorParamsAs1DForOutWhenUnconnected=off
  wires:
  AND/1 -> Out1/1
  In1/1 -> AND/2
  ForceRungInFalseRead/1(Out1) -> NOT/1
  NOT/1 -> AND/1

== system fukt_test/PLC Controller Suite/__Logic/Fukt sampling/Fuktmätare sampling/__Logic/TON/__CoreVarRead ==
  DataRead : DataStoreRead  DataStoreName=xxx_PLC_VAR_Fukt_periodicity  IndexOptions=Index vector (dialog)  Indices=1  OutputSizes=1
  y : Outport  VectorParamsAs1DForOutWhenUnconnected=off
  wires:
  DataRead/1 -> y/1

== system fukt_test/PLC Controller Suite/__Logic/Fukt sampling/Fuktmätare sampling/__Logic/TON1/BlockEnableRead ==
  __CoreLabelRead : Subsystem  Tag=CoreVarReadBlock  DisableCoverage=on  TreatAsAtomicUnit=on  mask{PLCBlockType=CoreLabelRead}
      mask init:
      | slplc.callbacks.initRoutineLabelRead(gcb);
      mask Help: web([docroot '/plccoder/ref/__corelabelread' '.html']);
      mask DialogControl PLCBlockTitle Prompt: Core Label Read
  Out1 : Outport  VectorParamsAs1DForOutWhenUnconnected=off
  wires:
  __CoreLabelRead/1(Out1) -> Out1/1
